simulink model "HVDCScan"  (R2025b)
settings: Solver=VariableStepAuto  StartTime=0.0  StopTime=Tsim  FixedStep=Ts  RelTol=1e-3
PreLoadFcn:
  | HVDCParameters
undefined symbols (not defined in the file): Connection1, Connection2, Connection3, DiscIntNeverNeededParam, ee_sli_rtmsupport, frt, gcbh, grid, HVDC, line, lvrt, pll, pmsm, scan, time, Ts, Vdcs0, windController, windTransformer, windTurbine
libraries: nesl_utility x36, fl_lib x24, ee_lib x18, eeGeneralControl x6, eeTransforms x3, simulink x1
(part 2 of 2)

== system HVDCScan/HVDC Cable (120 km)/Idcpr ==
  Current Sensor : fl_lib/Electrical/Electrical Sensors/Current Sensor
  PS-Simulink Converter : nesl_utility/PS-Simulink Converter  PhysicalDomain=network_engine_domain  SubClassName=ps_output  LeftPortType=input  RightPortType=output  PseudoPeriodic=off  Frequencies=[]  VectorFormat=1-D array  Unit=A  AffineConversion=off
  + : PMIOPort  Side=Left
  - : PMIOPort  Port=2  Side=Right
  i : Outport
  wires:
  PS-Simulink Converter/1 -> i/1
  connections:
  PS-Simulink Converter/LConn1 -- Current Sensor/RConn1
  Current Sensor/LConn1 -- +/RConn1
  -/RConn1 -- Current Sensor/RConn2

== system HVDCScan/HVDC Cable (120 km)/Idcps ==
  Current Sensor : fl_lib/Electrical/Electrical Sensors/Current Sensor
  PS-Simulink Converter : nesl_utility/PS-Simulink Converter  PhysicalDomain=network_engine_domain  SubClassName=ps_output  LeftPortType=input  RightPortType=output  PseudoPeriodic=off  Frequencies=[]  VectorFormat=1-D array  Unit=A  AffineConversion=off
  + : PMIOPort  Side=Left
  - : PMIOPort  Port=2  Side=Right
  i : Outport
  wires:
  PS-Simulink Converter/1 -> i/1
  connections:
  -/RConn1 -- Current Sensor/RConn2
  Current Sensor/LConn1 -- +/RConn1
  PS-Simulink Converter/LConn1 -- Current Sensor/RConn1

== system HVDCScan/HVDC Cable (120 km)/Vdcnr ==
  PS-Simulink Converter : nesl_utility/PS-Simulink Converter  PhysicalDomain=network_engine_domain  SubClassName=ps_output  LeftPortType=input  RightPortType=output  PseudoPeriodic=off  Frequencies=[]  VectorFormat=1-D array  Unit=V  AffineConversion=off
  Voltage Sensor : fl_lib/Electrical/Electrical Sensors/Voltage Sensor
  + : PMIOPort  Side=Left
  - : PMIOPort  Port=2  Side=Right
  v : Outport
  wires:
  PS-Simulink Converter/1 -> v/1
  connections:
  PS-Simulink Converter/LConn1 -- Voltage Sensor/RConn1
  Voltage Sensor/RConn2 -- -/RConn1
  Voltage Sensor/LConn1 -- +/RConn1

== system HVDCScan/HVDC Cable (120 km)/Vdcns ==
  PS-Simulink Converter : nesl_utility/PS-Simulink Converter  PhysicalDomain=network_engine_domain  SubClassName=ps_output  LeftPortType=input  RightPortType=output  PseudoPeriodic=off  Frequencies=[]  VectorFormat=1-D array  Unit=V  AffineConversion=off
  Voltage Sensor : fl_lib/Electrical/Electrical Sensors/Voltage Sensor
  + : PMIOPort  Side=Left
  - : PMIOPort  Port=2  Side=Right
  v : Outport
  wires:
  PS-Simulink Converter/1 -> v/1
  connections:
  Voltage Sensor/LConn1 -- +/RConn1
  Voltage Sensor/RConn2 -- -/RConn1
  PS-Simulink Converter/LConn1 -- Voltage Sensor/RConn1

== system HVDCScan/HVDC Cable (120 km)/Vdcpr ==
  PS-Simulink Converter : nesl_utility/PS-Simulink Converter  PhysicalDomain=network_engine_domain  SubClassName=ps_output  LeftPortType=input  RightPortType=output  PseudoPeriodic=off  Frequencies=[]  VectorFormat=1-D array  Unit=V  AffineConversion=off
  Voltage Sensor : fl_lib/Electrical/Electrical Sensors/Voltage Sensor
  + : PMIOPort  Side=Left
  - : PMIOPort  Port=2  Side=Right
  v : Outport
  wires:
  PS-Simulink Converter/1 -> v/1
  connections:
  Voltage Sensor/LConn1 -- +/RConn1
  Voltage Sensor/RConn2 -- -/RConn1
  PS-Simulink Converter/LConn1 -- Voltage Sensor/RConn1

== system HVDCScan/HVDC Cable (120 km)/Vdcps ==
  PS-Simulink Converter : nesl_utility/PS-Simulink Converter  PhysicalDomain=network_engine_domain  SubClassName=ps_output  LeftPortType=input  RightPortType=output  PseudoPeriodic=off  Frequencies=[]  VectorFormat=1-D array  Unit=V  AffineConversion=off
  Voltage Sensor : fl_lib/Electrical/Electrical Sensors/Voltage Sensor
  + : PMIOPort  Side=Left
  - : PMIOPort  Port=2  Side=Right
  v : Outport
  wires:
  PS-Simulink Converter/1 -> v/1
  connections:
  PS-Simulink Converter/LConn1 -- Voltage Sensor/RConn1
  Voltage Sensor/RConn2 -- -/RConn1
  Voltage Sensor/LConn1 -- +/RConn1

== system HVDCScan/HVDC STATION  (ST2)/Subsystem3 ==
  Vabc1 : Inport
  Vabc : Inport  Port=2
  Vref : Inport  Port=3
  F : Inport  Port=4
  F1 : InportShadow  Port=4
  Subsystem1 : Subsystem  ReferencedSubsystem=WFController  Kpv=offshoregfm.kvp  Kiv=offshoregfm.kvi  Kpicd=offshoregfm.kip  Kiicd=offshoregfm.kii  Kpicq=offshoregfm.kip  Kiicq=offshoregfm.kii  mVAbase=base.mVA  frequency=Grid.frequency  zBase=base.z  iMax=offshoregfm.Imax  L=HVDC.L/5  Kv=base.kV1
      settings: PortSchema="{\"entries\":[{\"content\":{\"sides\":[{\"content\":{\"connectorIds\":[\"In1\"]},\"type\":\"ConnectorPlacement.EquallySpacedRectSide\",\"uuid\":\"46af9a47-930e-4d26-bbce-c3520b6c2749\"},{\"content\":{\"connectorIds\":[\"Out1\"],\"side\":\"RIGHT\"},\"type\":\"ConnectorPlacement.EquallySpacedRectSide\",\"uuid\":\"6339fe7c-3981-41e7-9f19-cda16be41a14\"},{\"content\":{\"side\":\"TOP\"},\"type\":\"ConnectorPlacement.EquallySpacedRectSide\",\"uuid\":\"d1729033-563f-49aa-8053-bb4cbe37e0ab\"},{\"content\":{\"connectorIds\":[\"In2\",\"In3\"],\"side\":\"BOTTOM\"},\"type\":\"ConnectorPlacement.EquallySpacedRectSide\",\"uuid\":\"30ea6182-355c-4132-b992-4839827195ad\"}]},\"type\":\"ConnectorPlacement.EquallySpacedConnector\",\"uuid\":\"fc0bd660-6248-4e50-8baf-5497ce638304\"}],\"packageUris\":[\"http://schema.mathworks.com/mf0/Connector/R2020b\"],\"version\":\"1.0\"}"
  Subsystem2 : Subsystem  ReferencedSubsystem=WFController  Kpv=offshoregfm.kvp  Kiv=offshoregfm.kvi  Kpicd=offshoregfm.kip  Kiicd=offshoregfm.kii  Kpicq=offshoregfm.kip  Kiicq=offshoregfm.kii  mVAbase=base.mVA  frequency=Grid.frequency  zBase=base.z  iMax=offshoregfm.Imax  L=HVDC.L/5  Kv=base.kV1
      settings: PortSchema="{\"entries\":[{\"content\":{\"sides\":[{\"content\":{\"connectorIds\":[\"In1\"]},\"type\":\"ConnectorPlacement.EquallySpacedRectSide\",\"uuid\":\"46af9a47-930e-4d26-bbce-c3520b6c2749\"},{\"content\":{\"connectorIds\":[\"Out1\"],\"side\":\"RIGHT\"},\"type\":\"ConnectorPlacement.EquallySpacedRectSide\",\"uuid\":\"6339fe7c-3981-41e7-9f19-cda16be41a14\"},{\"content\":{\"side\":\"TOP\"},\"type\":\"ConnectorPlacement.EquallySpacedRectSide\",\"uuid\":\"d1729033-563f-49aa-8053-bb4cbe37e0ab\"},{\"content\":{\"connectorIds\":[\"In2\",\"In3\"],\"side\":\"BOTTOM\"},\"type\":\"ConnectorPlacement.EquallySpacedRectSide\",\"uuid\":\"30ea6182-355c-4132-b992-4839827195ad\"}]},\"type\":\"ConnectorPlacement.EquallySpacedConnector\",\"uuid\":\"fc0bd660-6248-4e50-8baf-5497ce638304\"}],\"packageUris\":[\"http://schema.mathworks.com/mf0/Connector/R2020b\"],\"version\":\"1.0\"}"
  Vref1 : InportShadow  Port=3
  VabcRef : Outport
  VabcRef1 : Outport  Port=2
  wires:
  Vabc/1 -> Subsystem1/1
  Vref/1 -> Subsystem1/3
  F/1 -> Subsystem1/2
  Vabc1/1 -> Subsystem2/1
  F1/1 -> Subsystem2/2
  Vref1/1 -> Subsystem2/3
  Subsystem1/1 -> VabcRef/1
  Subsystem2/1 -> VabcRef1/1

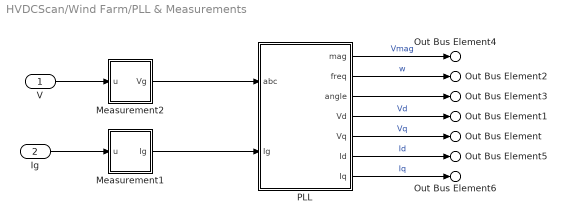
== system HVDCScan/Wind Farm/PLL & Measurements ==
  V : Inport
  Ig : Inport  Port=2
  Measurement1 : Subsystem
  Measurement2 : Subsystem
  PLL : Subsystem
  Out Bus Element : Outport  PortName=Vbus  Element=Vq
  Out Bus Element1 : Outport  PortName=Vbus  Element=Vd
  Out Bus Element2 : Outport  PortName=Vbus  Element=w
  Out Bus Element3 : Outport  PortName=Vbus  Element=Theta
  Out Bus Element4 : Outport  PortName=Vbus  Element=Vmag
  Out Bus Element5 : Outport  PortName=Vbus  Element=Id
  Out Bus Element6 : Outport  PortName=Vbus  Element=Iq
  wires:
  V/1 -> Measurement2/1(u)
  PLL/2(freq) -> Out Bus Element2/1  "w"
  PLL/5(Vq) -> Out Bus Element/1  "Vq"
  PLL/3(angle) -> Out Bus Element3/1
  PLL/4(Vd) -> Out Bus Element1/1  "Vd"
  Measurement2/1(Vg) -> PLL/1(abc)
  PLL/1(mag) -> Out Bus Element4/1  "Vmag"
  Measurement1/1(Ig) -> PLL/2(Ig)
  Ig/1 -> Measurement1/1(u)
  PLL/7(Iq) -> Out Bus Element6/1  "Iq"
  PLL/6(Id) -> Out Bus Element5/1  "Id"

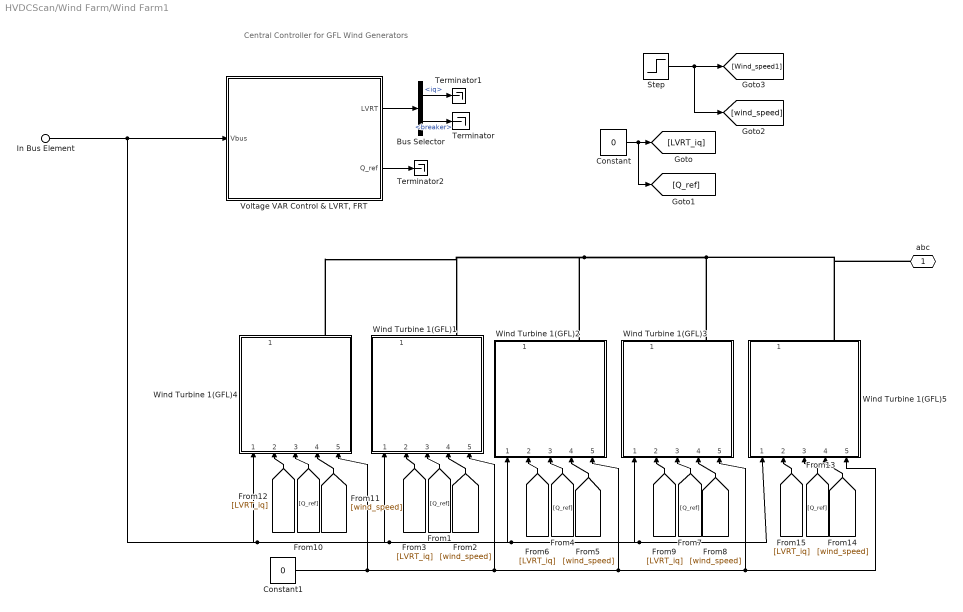
== system HVDCScan/Wind Farm/Wind Farm1 ==
  note: Central Controller for GFL Wind Generators
  In Bus Element : Inport  PortName=Vbus
  Bus Selector : BusSelector  OutputSignals=iq,breaker
  Constant : Constant  Value=0
  Constant1 : Constant  Value=0
  Step : Step  Time=time.renewablevariation  Before=11  After=10  SampleTime=Ts
  Terminator : Terminator
  Terminator1 : Terminator
  Terminator2 : Terminator
  "Voltage VAR Control & LVRT, FRT" : Subsystem
      mask Display: image('$imagefile'); % Use "Edit Image" on toolstrip to change.
  Wind Turbine 1(GFL){1..5} (5 alike) : Subsystem  ReferencedSubsystem=WindGFLMpp  p=pmsm.p  psim=pmsm.psim  Rs=pmsm.rs  Ld=pmsm.ld  Lq=pmsm.lq  Kdip_sm=pmsm.ld*pmsm.alpha  Kdii_sm=pmsm.rs*pmsm.alpha  Kqip_sm=pmsm.lq*pmsm.alpha  Kqii_sm=pmsm.rs*pmsm.alpha  airDensity=windTurbine.airDensity  turbineRadius=windTurbine.turbineRadius  pitch=windTurbine.pitch  TSR=windTurbine.TSR  cp=windTurbine.cp  wt=0.01  rt=0.01  Inertia=windTurbine.inertia  Kp_dc=windController.kpv  Ki_dc=windController.kiv  Kdpi_g=windController.kpic  Kdii_g=windController.kiic  Kqpi_g=windController.kpic  Kqii_g=windController.kiic  blk=Disabled  slop=0  tst=0
  abc : PMIOPort  Side=Right
  wires:
  Bus Selector/2 -> Terminator/1  "<breaker>"
  "Voltage VAR Control & LVRT, FRT"/1(LVRT) -> Bus Selector/1
  [LVRT_iq] -> Wind Turbine 1(GFL)1/2
  [wind_speed] -> Wind Turbine 1(GFL)1/4
  [Q_ref] -> Wind Turbine 1(GFL)1/3
  Step/1 -> [Wind_speed1], [wind_speed]
  Constant/1 -> [Q_ref], [LVRT_iq]
  Bus Selector/1 -> Terminator1/1  "<iq>"
  "Voltage VAR Control & LVRT, FRT"/2(Q_ref) -> Terminator2/1
  [LVRT_iq] -> Wind Turbine 1(GFL)2/2
  [Q_ref] -> Wind Turbine 1(GFL)2/3
  [wind_speed] -> Wind Turbine 1(GFL)2/4
  [Q_ref] -> Wind Turbine 1(GFL)3/3
  [wind_speed] -> Wind Turbine 1(GFL)3/4
  [LVRT_iq] -> Wind Turbine 1(GFL)3/2
  In Bus Element/1 -> Wind Turbine 1(GFL)5/1, Wind Turbine 1(GFL)3/1, Wind Turbine 1(GFL)2/1, Wind Turbine 1(GFL)1/1, Wind Turbine 1(GFL)4/1, "Voltage VAR Control & LVRT, FRT"/1(Vbus)
  [LVRT_iq] -> Wind Turbine 1(GFL)4/2
  [Q_ref] -> Wind Turbine 1(GFL)4/3
  [wind_speed] -> Wind Turbine 1(GFL)4/4
  [LVRT_iq] -> Wind Turbine 1(GFL)5/2
  [Q_ref] -> Wind Turbine 1(GFL)5/3
  [wind_speed] -> Wind Turbine 1(GFL)5/4
  Constant1/1 -> Wind Turbine 1(GFL)5/5, Wind Turbine 1(GFL)3/5, Wind Turbine 1(GFL)2/5, Wind Turbine 1(GFL)1/5, Wind Turbine 1(GFL)4/5
  connections:
  Wind Turbine 1(GFL)3/RConn1 -- abc/RConn1 -- Wind Turbine 1(GFL)5/RConn1 -- Wind Turbine 1(GFL)2/RConn1 -- Wind Turbine 1(GFL)4/RConn1 -- Wind Turbine 1(GFL)1/RConn1

== system HVDCScan/Wind Farm/PLL & Measurements/Measurement1 ==
  u : Inport
  Low-Pass Filter (Discrete or Continuous) : eeGeneralControl/Low-Pass Filter (Discrete or Continuous)  K=1  T=1e-4  B=inf  A=-inf  init_option=Inherited from block input  x0=0  Ts=-1
  Ig : Outport
  wires:
  u/1 -> Low-Pass Filter (Discrete or Continuous)/1
  Low-Pass Filter (Discrete or Continuous)/1 -> Ig/1

== system HVDCScan/Wind Farm/PLL & Measurements/Measurement2 ==
  u : Inport
  Low-Pass Filter (Discrete or Continuous) : eeGeneralControl/Low-Pass Filter (Discrete or Continuous)  K=1  T=1e-4  B=inf  A=-inf  init_option=Inherited from block input  x0=0  Ts=-1
  Vg : Outport
  wires:
  u/1 -> Low-Pass Filter (Discrete or Continuous)/1
  Low-Pass Filter (Discrete or Continuous)/1 -> Vg/1

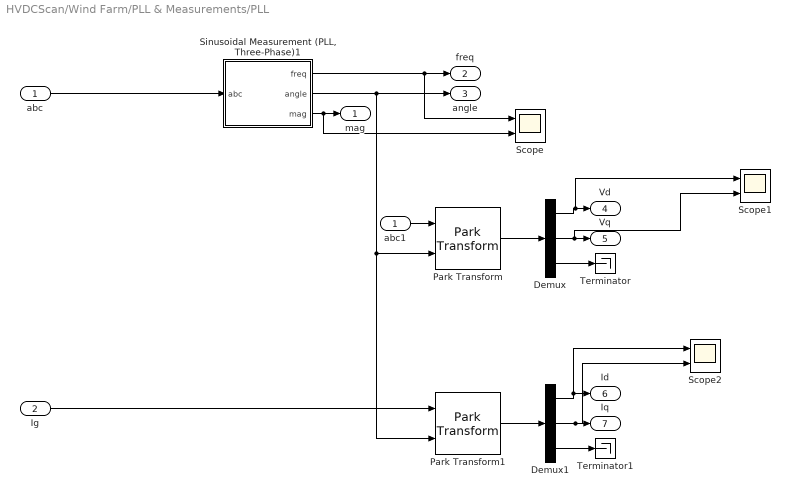
== system HVDCScan/Wind Farm/PLL & Measurements/PLL ==
  abc : Inport
  Ig : Inport  Port=2
  Demux : Demux  Outputs=3
  Demux1 : Demux  Outputs=3
  Park Transform : eeTransforms/Park Transform  AxisAlignment=Q-axis  PowerInvariant=off
  Park Transform1 : eeTransforms/Park Transform  AxisAlignment=Q-axis  PowerInvariant=off
  Scope : Scope  NumInputPorts=2
      settings: ActiveDisplayYMinimum=59.96953  ActiveDisplayYMaximum=60.08324
  Scope1 : Scope  NumInputPorts=2
      settings: ActiveDisplayYMinimum=-0.13188  ActiveDisplayYMaximum=1.18695  DataLoggingVariableName=ScopeData2
  Scope2 : Scope  NumInputPorts=2
      settings: ActiveDisplayYMinimum=-0.23524  ActiveDisplayYMaximum=1.13511  DataLoggingVariableName=ScopeData3
  "Sinusoidal Measurement (PLL, Three-Phase)1" : Subsystem  LoadFcn=ee_sli_rtmsupport( 'loadfcn', gcbh );  mask(Sinusoidal Measurement (PLL, Three-Phase)){Kp_LF=pll.kp, Ki_LF=pll.ki, F0=grid.frequency, Theta0=0, Ts=Ts}
      mask prompts: Kp_LF "physmod:ee:library:comments:control:eeSinusoidalMeasurement:LoopFilterProportionalGain_MP"; Ki_LF "physmod:ee:library:comments:control:eeSinusoidalMeasurement:LoopFilterIntegralGain_MP"; F0 "physmod:ee:library:comments:control:eeSinusoidalMeasurement:InitialFrequencyHz_MP"; Theta0 "physmod:ee:library:comments:control:eeSinusoidalMeasurement:InitialPhaseAnglerad_MP"; Ts "physmod:ee:library:comments:control:eeSinusoidalMeasurement:SampleTime1ForInherited_MP"
      mask help: physmod:ee:library:comments:control:eeSinusoidalMeasurement:SinusoidalPowerMeasurementPLLThreePhase_MD
      mask init:
      | timeDomain = ee.mask.initializeThreePhaseSinusoidalMeasurementPLL(Ts);
      settings: CopyFcn=ee_sli_rtmsupport( 'copyfcn', gcbh );  DeleteFcn=ee_sli_rtmsupport( 'deletefcn', gcbh );  ModelCloseFcn=ee_sli_rtmsupport( 'modelclosefcn', gcbh );  PostSaveFcn=ee_sli_rtmsupport( 'postsavefcn', gcbh );  PreCopyFcn=ee_sli_rtmsupport( 'precopyfcn', gcbh );  OpenFcn=ee_sli_rtmsupport( 'openfcn', gcbh );  CloseFcn=ee_sli_rtmsupport( 'closefcn', gcbh );  PreDeleteFcn=ee_sli_rtmsupport( 'predeletefcn', gcbh );
      settings: LibrarySourceBlock=|
      | ee_sl_lib/Measurements/Sinusoidal Measurement
      | (PLL, Three-Phase)
      mask Help: web(nesl_help(gcbh))
      mask TypeOptions Ts:
      | Angle/Integrator with
      | Wrapped State
      | (Discrete or Continuous)/Ts | PI/Integrator
      | (Discrete or Continuous)/Ts | Moving Average
      | (Variable Frequency)/Ts | Low-Pass Filter
      | (Discrete or Continuous)/Ts
      mask DialogControl Kp_LF Prompt: Loop filter proportional gain
      mask DialogControl Ki_LF Prompt: Loop filter integral gain
      mask DialogControl F0 Prompt: Initial frequency (Hz)
      mask DialogControl Theta0 Prompt: Initial phase angle (rad)
      mask DialogControl Ts Prompt: Sample time (-1 for inherited)
      mask Display: ee.mask.drawThreePhaseSinusoidalMeasurementPLL;
  Terminator : Terminator
  Terminator1 : Terminator
  abc1 : InportShadow
  mag : Outport
  freq : Outport  Port=2
  angle : Outport  Port=3
  Vd : Outport  Port=4
  Vq : Outport  Port=5
  Id : Outport  Port=6
  Iq : Outport  Port=7
  wires:
  Demux/3 -> Terminator/1
  Park Transform/1 -> Demux/1
  Demux/1 -> Scope1/1, Vd/1
  Demux/2 -> Scope1/2, Vq/1
  "Sinusoidal Measurement (PLL, Three-Phase)1"/3(mag) -> Scope/2, mag/1
  "Sinusoidal Measurement (PLL, Three-Phase)1"/2(angle) -> angle/1, Park Transform/2, Park Transform1/2
  Ig/1 -> Park Transform1/1
  Demux1/2 -> Scope2/2, Iq/1
  Park Transform1/1 -> Demux1/1
  Demux1/1 -> Scope2/1, Id/1
  Demux1/3 -> Terminator1/1
  abc1/1 -> Park Transform/1
  abc/1 -> "Sinusoidal Measurement (PLL, Three-Phase)1"/1(abc)
  "Sinusoidal Measurement (PLL, Three-Phase)1"/1(freq) -> Scope/1, freq/1

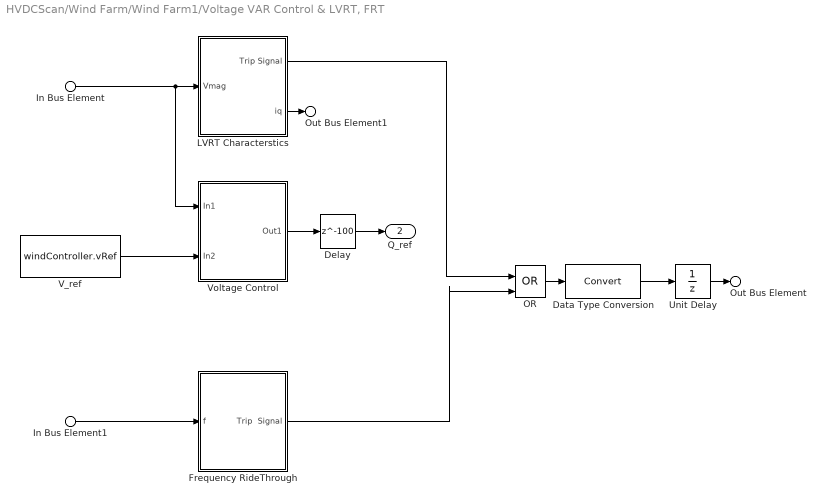
== system HVDCScan/Wind Farm/Wind Farm1/Voltage VAR Control & LVRT, FRT ==
  In Bus Element : Inport  PortName=Vbus  Element=Vmag
  In Bus Element1 : Inport  PortName=Vbus  Element=w
  Data Type Conversion : DataTypeConversion  RndMeth=Nearest  SaturateOnIntegerOverflow=off
  Delay : Delay  DelayLength=100
  Frequency RideThrough : Subsystem
  LVRT Characterstics : Subsystem
  OR : Logic  Operator=OR  IconShape=distinctive  AllPortsSameDT=off  OutDataTypeStr=boolean
  Unit Delay : UnitDelay  SampleTime=-1  HasFrameUpgradeWarning=on
  V_ref : Constant  Value=windController.vRef  SampleTime=Ts
  Voltage Control : Subsystem
  Out Bus Element : Outport  PortName=LVRT  Element=breaker
  Out Bus Element1 : Outport  PortName=LVRT  Element=iq
  Q_ref : Outport  Port=2
  wires:
  In Bus Element/1 -> LVRT Characterstics/1(Vmag), Voltage Control/1(In1)
  LVRT Characterstics/2(iq) -> Out Bus Element1/1
  V_ref/1 -> Voltage Control/2(In2)
  Voltage Control/1(Out1) -> Delay/1
  OR/1 -> Data Type Conversion/1
  LVRT Characterstics/1(Trip Signal) -> OR/1
  In Bus Element1/1 -> Frequency RideThrough/1(f)
  Data Type Conversion/1 -> Unit Delay/1
  Frequency RideThrough/1(Trip  Signal) -> OR/2
  Unit Delay/1 -> Out Bus Element/1
  Delay/1 -> Q_ref/1

== system HVDCScan/Wind Farm/PLL & Measurements/PLL/Sinusoidal Measurement (PLL, Three-Phase)1 ==
  note: Loop Filter (LF)
  note: Voltage-controlled oscillator (VCO)
  abc : Inport  PortDimensions=3  SampleTime=Ts
  Angle : Subsystem
  Low-Pass Filter (Discrete or Continuous) : eeGeneralControl/Low-Pass Filter (Discrete or Continuous)  K=1/2/pi  T=1e-3  B=inf  A=-inf  init_option=Specify as parameter  x0=F0  Ts=Ts
      settings: LibrarySourceBlock=|
      | eeSinusoidalMeasurementV2/Sinusoidal Measurement
      | (PLL, Three-Phase)/Low-Pass Filter
      | (Discrete or Continuous)
  Moving Average (Variable Frequency) : eeGeneralControl/Moving Average (Variable Frequency)  VariantControl=Variant1  LabelModeActiveChoice=Discrete  f0=F0  fmin=5  x0=0  BufferSize=8192  Ts=Ts
      settings: LibrarySourceBlock=|
      | eeSinusoidalMeasurementV2/Sinusoidal Measurement
      | (PLL, Three-Phase)/Moving Average
      | (Variable Frequency)
  PI : Subsystem
  Park Transform : eeTransforms/Park Transform  AxisAlignment=Q-axis  PowerInvariant=off
  Pythagorian Sum : Fcn  Expr=sqrt(u(1)^2+u(2)^2)
  Selector2 : Selector  InputPortWidth=3  IndexOptions=Index vector (dialog)  Indices=[2]  OutputSizes=1
  freq : Outport  VectorParamsAs1DForOutWhenUnconnected=off
  angle : Outport  Port=2  VectorParamsAs1DForOutWhenUnconnected=off
  mag : Outport  Port=3  VectorParamsAs1DForOutWhenUnconnected=off
  wires:
  Moving Average (Variable Frequency)/1 -> Selector2/1, Pythagorian Sum/1
  Selector2/1 -> PI/1(u)
  Low-Pass Filter (Discrete or Continuous)/1 -> freq/1, Moving Average (Variable Frequency)/1
  Angle/1(theta) -> angle/1, Park Transform/2
  PI/1(y) -> Angle/1(omega), Low-Pass Filter (Discrete or Continuous)/1
  Park Transform/1 -> Moving Average (Variable Frequency)/2
  Pythagorian Sum/1 -> mag/1
  abc/1 -> Park Transform/1

== system HVDCScan/Wind Farm/Wind Farm1/Voltage VAR Control & LVRT, FRT/Frequency RideThrough ==
  f : Inport
  Avoid Operation : Subsystem
  Discrete-Time Integrator1 : DiscreteIntegrator  ExternalReset=either  SampleTime=Ts  ICPrevOutput=DiscIntNeverNeededParam  ICPrevScaledInput=DiscIntNeverNeededParam
  Duration of f<fth : Lookup_n-D  NumberOfTableDimensions=1  BreakpointsForDimension1=(1+[-0.021,-0.02,0.02,0.021])*grid.frequency  Table=[1,0,0,1]  InterpMethod=Flat  InternalRulePriority=Speed  RndMeth=Simplest
  Frequency vs Trip time : Lookup_n-D  NumberOfTableDimensions=1  BreakpointsForDimension1=frt.frequency  Table=frt.time  InterpMethod=Flat  InternalRulePriority=Speed  RndMeth=Simplest
  GreaterThan : RelationalOperator  Operator=>  OutDataTypeStr=boolean  RndMeth=Simplest  InputSameDT=off
  Trip  Signal : Outport
  wires:
  Discrete-Time Integrator1/1 -> GreaterThan/1
  Frequency vs Trip time/1 -> GreaterThan/2
  GreaterThan/1 -> Trip  Signal/1
  Duration of f<fth/1 -> Discrete-Time Integrator1/2, Discrete-Time Integrator1/1
  Avoid Operation/1(f) -> Duration of f<fth/1, Frequency vs Trip time/1
  f/1 -> Avoid Operation/1(f_in)

== system HVDCScan/Wind Farm/Wind Farm1/Voltage VAR Control & LVRT, FRT/LVRT Characterstics ==
  Vmag : Inport
  Discrete-Time Integrator1 : DiscreteIntegrator  ExternalReset=either  SampleTime=Ts  ICPrevOutput=DiscIntNeverNeededParam  ICPrevScaledInput=DiscIntNeverNeededParam
  Duration of Vmag<Vth : Lookup_n-D  NumberOfTableDimensions=1  BreakpointsForDimension1=[0,.9,0.91,1.2]  Table=[1,1,0,0]  InterpMethod=Flat  InternalRulePriority=Speed  RndMeth=Simplest
  Gain1 : Gain  Gain=-1
  GreaterThan : RelationalOperator  Operator=>  OutDataTypeStr=boolean  RndMeth=Simplest  InputSameDT=off
  Saturation2 : Saturate  UpperLimit=1/8  LowerLimit=-1
  Vmag vs Trip time : Lookup_n-D  NumberOfTableDimensions=1  BreakpointsForDimension1=lvrt.voltage  Table=lvrt.time  InterpMethod=Flat  InternalRulePriority=Speed  RndMeth=Simplest
  Vmag vs iq : Lookup_n-D  NumberOfTableDimensions=1  BreakpointsForDimension1=lvrt.voltageiq  Table=lvrt.iq  InternalRulePriority=Speed  RndMeth=Simplest
  Trip Signal : Outport
  iq : Outport  Port=2
  wires:
  Duration of Vmag<Vth/1 -> Discrete-Time Integrator1/2, Discrete-Time Integrator1/1
  GreaterThan/1 -> Trip Signal/1
  Discrete-Time Integrator1/1 -> GreaterThan/1
  Vmag vs Trip time/1 -> GreaterThan/2
  Vmag vs iq/1 -> Saturation2/1
  Gain1/1 -> iq/1
  Saturation2/1 -> Gain1/1
  Vmag/1 -> Vmag vs iq/1, Vmag vs Trip time/1, Duration of Vmag<Vth/1

== system HVDCScan/Wind Farm/Wind Farm1/Voltage VAR Control & LVRT, FRT/Voltage Control ==
  In1 : Inport
  In2 : Inport  Port=2
  Constant2 : Constant  Value=0
  Gain : Gain  Gain=windController.mv
  Sum2 : Sum  Inputs=|+-
  Switch1 : Switch  Threshold=.9  SaturateOnIntegerOverflow=off  InputSameDT=off
  Out1 : Outport
  wires:
  Gain/1 -> Out1/1
  Sum2/1 -> Switch1/1
  Switch1/1 -> Gain/1
  In1/1 -> Sum2/2, Switch1/2
  Constant2/1 -> Switch1/3
  In2/1 -> Sum2/1

== system HVDCScan/Wind Farm/PLL & Measurements/PLL/Sinusoidal Measurement (PLL, Three-Phase)1/Angle ==
  omega : Inport
  Integrator with Wrapped State (Discrete or Continuous) : eeGeneralControl/Integrator with Wrapped State (Discrete or Continuous)  LabelModeActiveChoice=Discrete  WrappedStateUpperValue=2*pi  WrappedStateLowerValue=0  x0=Theta0  Ts=Ts
      settings: LibrarySourceBlock=|
      | eeSinusoidalMeasurementV2/Sinusoidal Measurement
      | (PLL, Three-Phase)/Angle/Integrator with
      | Wrapped State
      | (Discrete or Continuous)
  theta : Outport  VectorParamsAs1DForOutWhenUnconnected=off
  wires:
  Integrator with Wrapped State (Discrete or Continuous)/1 -> theta/1
  omega/1 -> Integrator with Wrapped State (Discrete or Continuous)/1

== system HVDCScan/Wind Farm/PLL & Measurements/PLL/Sinusoidal Measurement (PLL, Three-Phase)1/PI ==
  u : Inport
  Constant : Constant  Value=2*pi*F0  SampleTime=Ts
  Constant1 : Constant  Value=0  SampleTime=Ts
  Data Type Conversion Inherited : simulink/Signal Attributes/Data Type Conversion Inherited  ConvertRealWorld=Real World Value  DoSatur=off
  Gain : Gain  Gain=Kp_LF
  Gain1 : Gain  Gain=Ki_LF
  Integrator (Discrete or Continuous) : eeGeneralControl/Integrator (Discrete or Continuous)  LabelModeActiveChoice=Discrete  IntegratorMethod=Integration: Forward Euler  ExternalReset=level  LimitType=Anti-windup  B=inf  A=-inf  Ts=Ts
      settings: LibrarySourceBlock=|
      | eeSinusoidalMeasurementV2/Sinusoidal Measurement
      | (PLL, Three-Phase)/PI/Integrator
      | (Discrete or Continuous)
  Sum : Sum  Inputs=|++
  y : Outport  VectorParamsAs1DForOutWhenUnconnected=off
  wires:
  Constant/1 -> Data Type Conversion Inherited/2
  Data Type Conversion Inherited/1 -> Integrator (Discrete or Continuous)/3
  Gain1/1 -> Integrator (Discrete or Continuous)/1
  u/1 -> Gain1/1, Data Type Conversion Inherited/1, Gain/1
  Gain/1 -> Sum/1
  Integrator (Discrete or Continuous)/1 -> Sum/2
  Sum/1 -> y/1
  Constant1/1 -> Integrator (Discrete or Continuous)/2

== system HVDCScan/Wind Farm/Wind Farm1/Voltage VAR Control & LVRT, FRT/Frequency RideThrough/Avoid Operation ==
  f_in : Inport
  Constant : Constant  Value=grid.frequency  SampleTime=Ts
  Step : Step  Time=0.5  SampleTime=Ts
  Switch : Switch  Criteria=u2 > Threshold  SaturateOnIntegerOverflow=off  InputSameDT=off
  f : Outport
  wires:
  f_in/1 -> Switch/1
  Constant/1 -> Switch/3
  Step/1 -> Switch/2
  Switch/1 -> f/1
